simulink model "ThreePhaseFullyControlled"  (R2024b)
settings: Solver=VariableStepAuto  StartTime=0.0  StopTime=0.1  RelTol=1e-3
libraries: spsThyristorLib x6, spsVoltageMeasurementLib x5, spsCurrentMeasurementLib x2, spsGroundLib x1, spsSeriesRLCBranchLib x1, spsThreePhaseProgrammableVoltageSourceLib x1, sps_lib x1
settings Model: Creator=harsh  LastModifiedBy=harsh

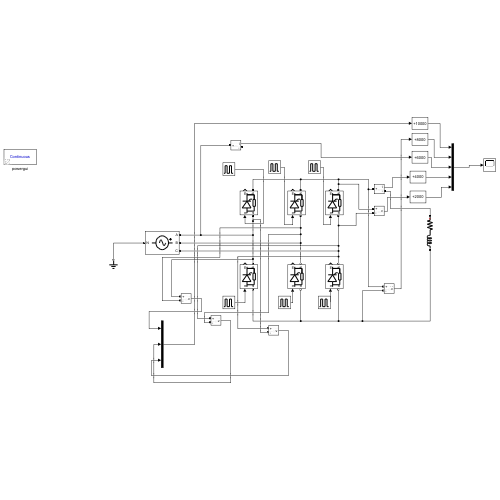
[thumbnail: Simulink's stored preview of the top-level diagram]
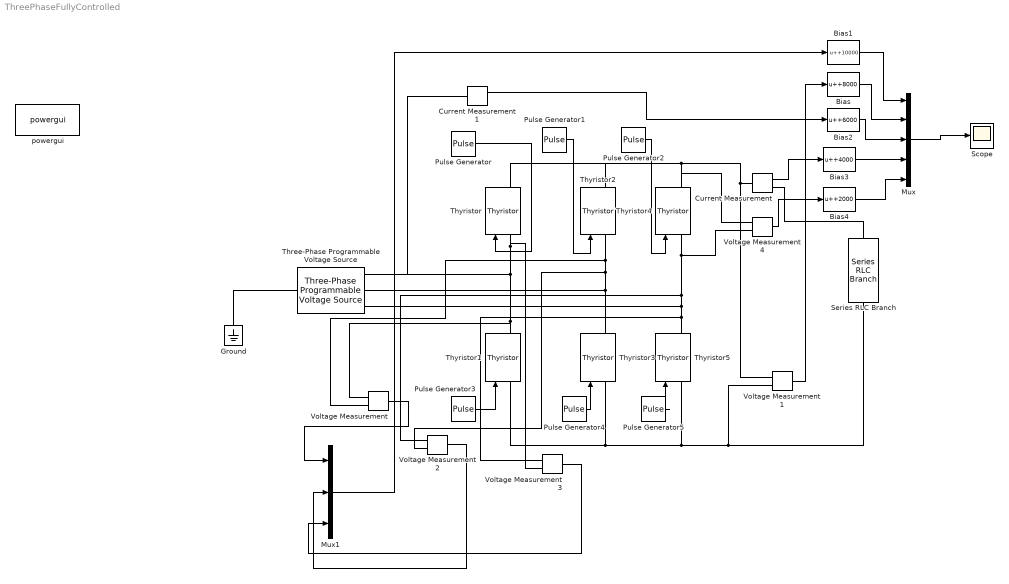
== system ThreePhaseFullyControlled ==
  Bias : Bias  Bias=+8000  SaturateOnIntegerOverflow=off
  Bias1 : Bias  Bias=+10000  SaturateOnIntegerOverflow=off
  Bias2 : Bias  Bias=+6000  SaturateOnIntegerOverflow=off
  Bias3 : Bias  Bias=+4000  SaturateOnIntegerOverflow=off
  Bias4 : Bias  Bias=+2000  SaturateOnIntegerOverflow=off
  Current Measurement : spsCurrentMeasurementLib/Current Measurement  PhasorSimulation=off  OutputType=Complex  PSBequivalent=0
  Current Measurement1 : spsCurrentMeasurementLib/Current Measurement  PhasorSimulation=off  OutputType=Complex  PSBequivalent=0
  Ground : spsGroundLib/Ground  LConnTagsString=a
  Mux : Mux  Inputs=5
  Mux1 : Mux  Inputs=3
  Pulse Generator : DiscretePulseGenerator  PulseType=Time based  Period=0.02  PulseWidth=5  PhaseDelay=0*0.02/360
  Pulse Generator1 : DiscretePulseGenerator  PulseType=Time based  Period=0.02  PulseWidth=5  PhaseDelay=(0+120)*0.02/360
  Pulse Generator2 : DiscretePulseGenerator  PulseType=Time based  Period=0.02  PulseWidth=5  PhaseDelay=(0+240)*0.02/360
  Pulse Generator3 : DiscretePulseGenerator  PulseType=Time based  Period=0.02  PulseWidth=5  PhaseDelay=(0+180)*0.02/360
  Pulse Generator4 : DiscretePulseGenerator  PulseType=Time based  Period=0.02  PulseWidth=5  PhaseDelay=(0+300)*0.02/360
  Pulse Generator5 : DiscretePulseGenerator  PulseType=Time based  Period=0.02  PulseWidth=5  PhaseDelay=(0+60)*0.02/360
  Scope : Scope
  Series RLC Branch : spsSeriesRLCBranchLib/Series RLC Branch  LConnTagsString=__new0  RConnTagsString=__new0  BranchType=RL  Resistance=1  Inductance=6*10^-3  SetiL0=off  InitialCurrent=0  Capacitance=1e-6  Setx0=off  InitialVoltage=0  Measurements=None
  Three-Phase Programmable Voltage Source : spsThreePhaseProgrammableVoltageSourceLib/Three-Phase Programmable Voltage Source  PositiveSequence=[400 0 50]  VariationEntity=None  VariationType=Table of time-amplitude pairs  VariationTypeAlt=Step  VariationStep=0.5  VariationRate=10  VariationMagnitude=0.3  VariationFrequency=2  VariationTiming=[1 2]  VariationPhaseA=off  Amplitudes=[1 0.8 1.2 1.0]  TimeValues=[0 0.1 0.15 0.2]  HarmonicGeneration=off  HarmonicA=[3 0.2 -25 0]  HarmonicB=[2 0.15 35 2]  Timing="[0.05  3]"  BusType=swing  Pref=0  Qref=0  Qmin=-inf  Qmax=inf
  Thyristor{,1..5} (6 alike) : spsThyristorLib/Thyristor  Ron=0.001  Lon=0  Vf=0.8  IC=0  Rs=500  Cs=250e-9  Measurements=on
  Voltage Measurement{,1..4} (5 alike) : spsVoltageMeasurementLib/Voltage Measurement  PhasorSimulation=off  OutputType=Complex  PSBequivalent=0
  powergui : sps_lib/powergui  Priority=1  SimulationMode=Continuous  SampleTime=50e-6  frequency=60  Iterations=50  frequencyindice=50  Pbase=100e6  ErrMax=1e-4  UnitsV=kV  UnitsW=MW  buscounter=0  FunctionMessages=off  echomessages=off  EnableUseOfTLC=off  CurrentSourceSwitches=off  DisableSnubberDevices=off  DisableRonSwitches=off  DisableVfSwitches=off  DisplayEquations=off  AutomaticDiscreteSolvers=off  SolverType=Tustin/Backward Euler (TBE)  Interpol=off  ExternalGateDelay=off  methode=off  Ts=100  x0status=blocks  SPID=on  SwTol=0  HookPort=off  NonlinearTolerance=1e-4  nMaxIteration=100  ContinueOnMaxIteration=off  RestoreLinks=warning  ResistiveCurrentMeasurement=off  Frange=[0:2:500]  Ylog=off  Xlog=on  ShowGrid=off  save=off  variable=ZData  structure=0  ZoomFFT=off  StartTime=0.0  cycles=1  DisplayStyle=1  fundamental=60  FreqAxis=off  MaxFrequency=1000  frequencyindicesteady=1  RmsSteady=1  display=off
  wires:
  Pulse Generator/1 -> Thyristor/1
  Pulse Generator1/1 -> Thyristor2/1
  Pulse Generator2/1 -> Thyristor4/1
  Pulse Generator3/1 -> Thyristor1/1
  Pulse Generator4/1 -> Thyristor3/1
  Pulse Generator5/1 -> Thyristor5/1
  Voltage Measurement/1 -> Mux1/1
  Mux/1 -> Scope/1
  Voltage Measurement2/1 -> Mux1/2
  Voltage Measurement3/1 -> Mux1/3
  Mux1/1 -> Bias1/1
  Bias1/1 -> Mux/1
  Voltage Measurement1/1 -> Bias/1
  Bias/1 -> Mux/2
  Current Measurement/1 -> Bias3/1
  Current Measurement1/1 -> Bias2/1
  Voltage Measurement4/1 -> Bias4/1
  Bias4/1 -> Mux/5
  Bias3/1 -> Mux/4
  Bias2/1 -> Mux/3
  connections:
  Thyristor/LConn1 -- Current Measurement1/LConn1 -- Three-Phase Programmable Voltage Source/RConn1 -- Voltage Measurement/LConn1 -- Thyristor1/RConn1 -- Voltage Measurement3/LConn2
  Thyristor2/LConn1 -- Voltage Measurement/LConn2 -- Voltage Measurement2/LConn2 -- Three-Phase Programmable Voltage Source/RConn2 -- Thyristor3/RConn1
  Thyristor4/LConn1 -- Voltage Measurement2/LConn1 -- Three-Phase Programmable Voltage Source/RConn3 -- Voltage Measurement3/LConn1 -- Thyristor5/RConn1 -- Voltage Measurement4/LConn2
  Current Measurement/RConn1 -- Series RLC Branch/LConn1
  Thyristor1/LConn1 -- Thyristor3/LConn1 -- Voltage Measurement1/LConn2 -- Series RLC Branch/RConn1 -- Thyristor5/LConn1
  Voltage Measurement1/LConn1 -- Voltage Measurement4/LConn1 -- Thyristor4/RConn1 -- Thyristor2/RConn1 -- Thyristor/RConn1 -- Current Measurement/LConn1
  Ground/LConn1 -- Three-Phase Programmable Voltage Source/LConn1
